simulink model "IEEE_9bus_4"  (Simulink 8.4)
settings: Solver=ode4  StartTime=0.0  StopTime=inf  FixedStep=Ts  RelTol=1e-3
PostLoadFcn:
  | Ts=25e-6;Rs=5*1.867;cs=1.4080e-004;
InitFcn:
  | Ts=25e-6;Rs=5*1.867;cs=1.4080e-004;
undefined symbols (not defined in the file): another_event_name, gcbh, my_event_name, sps_rtmsupport
libraries: spsVIMeasurementModel x36, powerlib x34, powerlib_meascontrol x18, rtlab x4, artemis x3, sps_avr x3
(part 1 of 3)
Description:
  | Model of a simple control system for use iin training.
settings Model: ARTEMISmethode_block_infos=$$__separator__$$IEEE_9bus_4/ARTEMIS Guide$$__separator__$$  Creator=Paul Baracos  LastModifiedBy=opal-user  BufferReuse=off
settings DataIOCC: SaveOutput=off  SaveTime=off  SignalLoggingName=sigsOut
settings OptimizationCC: BlockReduction=off  BooleanDataType=off  OptimizeBlockIOStorage=off  BufferReuse=off  GlobalBufferReuse=off  ExpressionFolding=off  ExpressionDepthLimit=128  LocalBlockOutputs=off  InitFltsAndDblsToZero=on
settings DebuggingCC: SaveWithParameterizedLinksMsg=none  SignalResolutionControl=TryResolveAllWithWarning  SolverPrmCheckMsg=none  MultiTaskDSMMsg=warning  MultiTaskCondExecSysMsg=none  StateNameClashWarn=none
settings HardwareCC: TargetUnknown=on
settings RTWCC: IncludeERTFirstTime=on
settings GRTTargetCC: TargetFcnLib=ansi_tfl_tmw.mat

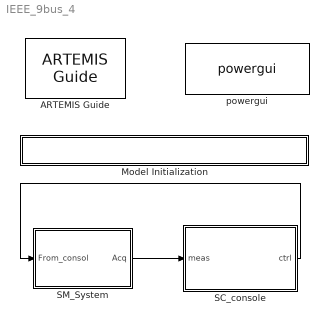
== system IEEE_9bus_4 ==
  ARTEMIS Guide : artemis/ARTEMIS/ARTEMIS Guide  Tag=FTSSmethode_opal_4hx0r99  Description=5.0_z1  lock=on  Ts=Ts  opt=art5  dyna=off  nb_perm=50  RT_fullcomp=off  ssn=off  ssn_itvc=off  ssn_ivic=off  ssn_ext=off  ssn_solver=Art5  ssn_impulse=off  ssn_quasimpulse=off  ssn_impulse_loop=2  paraExtinctionThy=off  Thy_Impulse=on  dtc=Off  dtc_opt=true impulse event detection  ao=on  simtype=off  ct_mac=off  lin_mov=off  lsp=[0.001 2]  spike_skip=Disabled  dtc_extra=1  dtc_sws=normal  dtc_pied=0.5  SPSRulesBlock=SPSRules  tre=on  ctmm=off  LF=off  dpl_type=ARTEMiS DPL  rlc_type=off  custom_type=off  para=off  ssn_ImpulseLoopBlockedStateUpdate=2  ssn_mov_iter_number=5  ssn_switch_iter_number=5
  Model Initialization : Subsystem  mask(Model Functions){InitFcnX=Ts=25e-6;Rs=5*1.867;cs=1.4080e-004;, prel=off, posl=on, inif=on, strf=off}
      mask prompts: InitFcnX "Initialisation"; prel "Preload Function"; posl "PostLoad Function"; inif "InitFcn"; strf "StartFcn"
      mask init:
      | currentBlock = gcb;
      | root = bdroot(currentBlock);
      | 
      | if ~strcmp(get_param(root,'BlockDiagramType'),'library')
      |     if prel==1
      |         set_param(root, 'PreLoadFcn', InitFcnX);
      |     else
      |         set_param(root, 'PreLoadFcn', '');
      |     end
      |     if inif==1
      |         set_param(root, 'InitFcn', InitFcnX);
      |     else
      |         set_param(root, 'InitFcn', '');
      |     end
      |     if strf==1
      |         set_param(root, 'StartFcn', InitFcnX);
      |     else
      |         set_param(root, 'StartFcn', '');
      |     end
      |     if posl==1
      |         set_param(root, 'PostLoadFcn', InitFcnX);
      |     else
      |         set_param(root, 'PostLoadFcn', '');
      |     end
      | end
      | 
      | pos = get_param(currentBlock, 'Position');
      | width = pos(3) - pos(1); height = pos(4) - pos(2);
      | txt = [ upper(root) '\n' '- InitFcn. . . . . '  get_param(root, 'InitFcn') ];
      settings: CopyFcn=set_param(gcb,'LinkStatus','none')
      mask Display: text(5, height*0.5, txt, 'horizontalAlignment', 'left', 'verticalAlignment', 'middle') ;
  SC_console : Subsystem
  SM_System : Subsystem
  powergui : powerlib/powergui  Priority=1  SimulationMode=Discrete  SolverType=Tustin  SampleTime=Ts  frequency=60  SPID=off  DisableSnubberDevices=off  DisableRonSwitches=off  DisableVfSwitches=off  SwTol=0  DisplayEquations=off  Interpol=off  methode=off  Ts=0  frequencyindice=60  Pbase=100e6  ErrMax=1e-4  Iterations=50  UnitsV=kV  UnitsW=MW  FunctionMessages=off  echomessages=off  HookPort=off  EnableUseOfTLC=off  x0status=steady  RestoreLinks=warning  ResistiveCurrentMeasurement=off  Frange=[0:2:500]  Ylog=off  Xlog=on  ShowGrid=off  save=off  variable=ZData  structure=0  ZoomFFT=on  StartTime=0.0  cycles=1  DisplayStyle=1  fundamental=60  FreqAxis=off  MaxFrequency=1000  frequencyindicesteady=1  RmsSteady=1  display=off
  wires:
  SC_console/1(ctrl) -> SM_System/1(From_consol)
  SM_System/1(Acq) -> SC_console/1(meas)

== system IEEE_9bus_4/Model Initialization ==

== system IEEE_9bus_4/SC_console ==
  note: System Setting
  note: Green for basic setting/scoping
  note: Orange for advanced setting/scoping
  note: System Scoping
  note: 7-Three-Phase Bus Transmission and Distribution System
  meas : Inport
  Breakers Control1 : Subsystem
  Fault Set1 : Subsystem  mask(fault set){Tacq=1, Tst=[0.5 0 10], Tdr=[0.1 0 10], Ftype=0:no fault, L1=off, L2=off, L3=off}
      mask prompts: Tacq "acquisition period"; Tst "fault start time set [Tst, Tst_var, Tst_pd]"; Tdr "fault duration set [Tst, Tst_var, Tst_pd]"; Ftype "fault_type"; L1 "Location 1"; L2 "Location 2"; L3 "Location 3"
      mask help:
      | output dimention: 8=1+3+3+1
      |
      | acquisition period, Tacq
      |
      | fault start time set [Tst, Tst_var, Tst_pd]
      | if Tst_var=0, fault starts at Tst
      | if Tst_var<>0, Tst varies from Tst to Tst+Tst_var, variation cycle is Tst_pd.
      |
      | fault duration set [Tdr, Tdr_var, Tdr_pd]
      | if Tdr_var=0, fault durstion is fixed, equal Tdr
      | if Tdr_var<>0, fault duration varies from Tdr to Tdr+Tdr_var, variation cycle is Tdr_pd.
      |
      | fault_type
      mask init:
      | switch Ftype
      |     case 1
      |         x='no fault';
      |     case 2
      | 	x='a fault';
      |     case 3
      | 	x='b fault';
      |     case 4
      | 	x='c fault';
      |     case 5
      | 	x='ab fault';
      |     case 6
      | 	x='ac fault';
      |     case 7
      | 	x='bc fault';
      |     case 8
      | 	x='abc gnd fault';
      | end
      mask TypeOptions Ftype: 0:no fault | 1:a fault | 2: b fault | 3:c fault | 4:ab fault | 5: ac fault | 6: bc fault | 7:abc-gnd fault
      mask Display: disp(x,Tacq)
  Help : artemis/Internal/Help  docfile=..\help\adgrid22_7bus_hvac.html
  Mux : Mux  Inputs=3
  OpComm1 : rtlab/OpComm  nbport=1  groupe_acq=1  subsys_rate=0  st=0  Synchronization=on  Interpolation=on  Threshold=1.0  Missed_Data=off  Sim_Time=off  Samples=off  dynSigOut=off  from_console=0  warning_done=off  writeOpCommFile=off  Offset=off
  SM_Select : Subsystem
  Subsystem : Subsystem
  www.opal-rt.com1 : artemis/Internal/www.opal-rt.com  SystemSampleTime=-1
  ctrl : Outport
  wires:
  meas/1 -> OpComm1/1
  Mux/1 -> ctrl/1
  Fault Set1/1(Out1) -> Mux/2
  Breakers Control1/1(BR_CTRL) -> Mux/1
  SM_Select/1(SM) -> Mux/3
  OpComm1/1 -> Subsystem/1(In3)

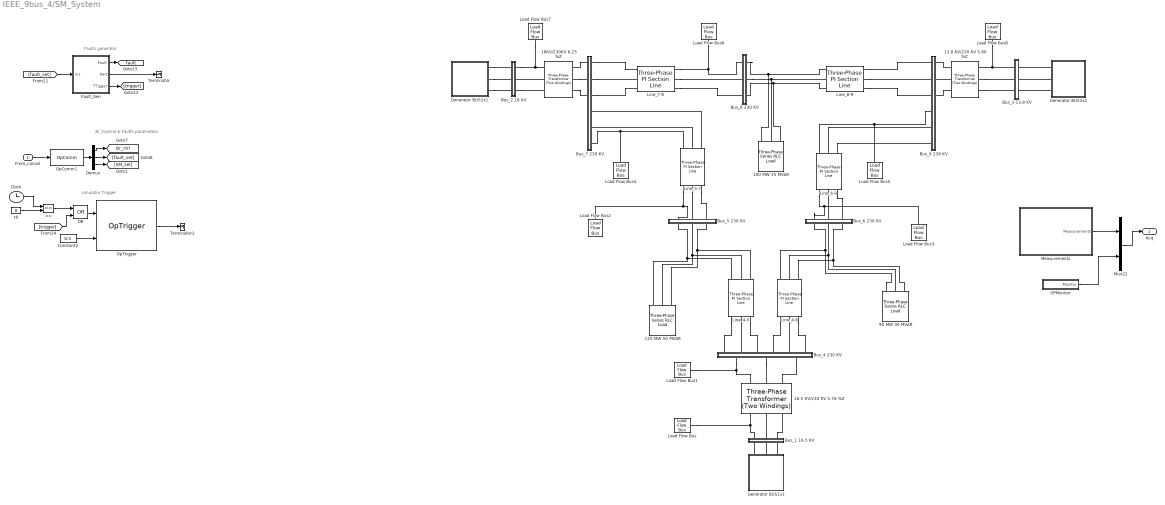
== system IEEE_9bus_4/SM_System ==
  note: Br_Control & Faults parameters
  note: Faults generator
  note: simulator Trigger
  From_consol : Inport
  100 MW 35 MVAR : powerlib/Elements/Three-Phase Series RLC Load  LConnTagsString=A|B|C  Configuration=Y (grounded)  NominalVoltage=(230000)*1.01601  NominalFrequency=60  ActivePower=100e6  InductivePower=35e6  CapacitivePower=0  Measurements=Branch voltages and currents  LoadType=constant PQ
  125 MW 50 MVAR : powerlib/Elements/Three-Phase Series RLC Load  LConnTagsString=A|B|C  Configuration=Y (grounded)  NominalVoltage=(230000)*0.996126  NominalFrequency=60  ActivePower=125e6  InductivePower=50e6  CapacitivePower=0  Measurements=Branch voltages and currents  LoadType=constant PQ
  13.8 KV/230 KV 5.86 %Z : powerlib/Elements/Three-Phase Transformer (Two Windings)  Winding1Connection=Yg  UNITS=pu  NominalPower=[ 128e6 , 60 ]  Winding1=[ 13.8e3 , 1e-6 , 0.0 ]  Winding2Connection=Yg  Winding2=[ 230e3 , 1e-6, 0.075008 ]  SetSaturation=off  Rm=inf  Lm=inf  Saturation=[ 0,0 ; 0.0024,1.2 ; 1.0,1.52 ]  Hysteresis=off  DataFile='hysteresis'  SetInitialFlux=off  InitialFluxes=[ 0.8 , -0.8 , 0.7 ]  Measurements=None  MoreParameters=off  BreakLoop=off  DataType=off  TransfoNumber=1
  "16.5 KV/230 KV 5.76 %Z     " : powerlib/Elements/Three-Phase Transformer (Two Windings)  Winding1Connection=Yg  UNITS=pu  NominalPower=[ 247.5e6 , 60 ]  Winding1=[ 16.5e3 , 1e-6, 0.0 ]  Winding2Connection=Yg  Winding2=[ 230e3 ,1e-6, 0.14256 ]  SetSaturation=off  Rm=inf  Lm=inf  Saturation=[ 0,0 ; 0.0024,1.2 ; 1.0,1.52 ]  Hysteresis=off  DataFile='hysteresis'  SetInitialFlux=off  InitialFluxes=[ 0.8 , -0.8 , 0.7 ]  Measurements=None  MoreParameters=off  BreakLoop=off  DataType=off  TransfoNumber=1
  18KV/230KV 6.25 %Z : powerlib/Elements/Three-Phase Transformer (Two Windings)  Winding1Connection=Yg  UNITS=pu  NominalPower=[ 192e6 , 60 ]  Winding1=[ 18e3 , 1e-6 , 0.0 ]  Winding2Connection=Yg  Winding2=[ 230e3 , 1e-6, 0.12 ]  SetSaturation=off  Rm=inf  Lm=inf  Saturation=[ 0,0 ; 0.0024,1.2 ; 1.0,1.52 ]  Hysteresis=off  DataFile='hysteresis'  SetInitialFlux=off  InitialFluxes=[ 0.8 , -0.8 , 0.7 ]  Measurements=None  MoreParameters=off  BreakLoop=off  DataType=off  TransfoNumber=1
  90 MW 30 MVAR : powerlib/Elements/Three-Phase Series RLC Load  LConnTagsString=A|B|C  Configuration=Y (grounded)  NominalVoltage=(230000)*1.01311  NominalFrequency=60  ActivePower=90e6  InductivePower=30e6  CapacitivePower=0  Measurements=Branch voltages and currents  LoadType=constant PQ
  == : RelationalOperator  Operator===  InputSameDT=on
  Bus_1 16.5 KV : Subsystem  DialogController=POWERSYS.PowerSysDialog  LoadFcn=sps_rtmsupport('LoadFcn',gcbh);  StartFcn=sps_rtmsupport('StartFcn',gcbh);  StopFcn=sps_rtmsupport('StopFcn',gcbh);  mask(Three-Phase VI Measurement){VoltageMeasurement=phase-to-phase, SetLabelV=on, LabelV=Vabc_1, Vpu=off, VpuLL=off, CurrentMeasurement=yes, SetLabelI=on, LabelI=Iabc_1, Ipu=off, Pbase=100e6, Vbase=16.5e3, OutputType=Complex, PhasorSimulation=off, PSBequivalent=0}
      mask prompts: VoltageMeasurement "Voltage measurement"; SetLabelV "Use a label"; LabelV "Signal label  (use a From block to collect this signal)"; Vpu "Voltages in pu,  based on peak value of nominal phase-to-ground voltage"; VpuLL "Voltages in pu,  based on peak value of nominal phase-to-phase  voltage"; CurrentMeasurement "Current measurement"; SetLabelI "Use a label"; LabelI "Signal label  (use a From block to collect this signal)"; Ipu "Currents in pu"; Pbase "Base power ( VA 3 phase)"; Vbase "Nominal voltage used for pu measurement (Vrms phase-phase) :"; OutputType "Output signals in:"; PhasorSimulation "Phasor simulation (internal use)"; PSBequivalent "Equivalent circuit (internal use)"
      mask help:
      | Ideal three-phase voltage and current measurements.
      |
      | The block can output the voltages and currents in per unit values or in volts and amperes.
      mask init:
      | block = gcb;
      | Kv=1;
      | Ki=1;
      | [Kv,Ki] = powericon('ThreePhaseVIMeasurementParam',block,Vpu,VpuLL,Ipu,Vbase,Pbase,PhasorSimulation,OutputType);
      | powericon('ThreePhaseVIMeasurementCback',block);
      | power_initmask();
      settings: CopyFcn=sps_rtmsupport('CopyFcn',gcbh); powericon('ThreePhaseVIMeasurementCopy',gcb)  DeleteFcn=sps_rtmsupport('DeleteFcn',gcbh);  UndoDeleteFcn=sps_rtmsupport('UndoDeleteFcn',gcbh);  ModelCloseFcn=sps_rtmsupport('ModelCloseFcn',gcbh);  PreSaveFcn="sps_rtmsupport('PreSaveFcn',gcbh);  set_param(gcb,'LinkStatus','restore')"  PostSaveFcn=sps_rtmsupport('PostSaveFcn',gcbh);  NameChangeFcn=sps_rtmsupport('NameChangeFcn',gcbh);  PreCopyFcn=sps_rtmsupport('PreCopyFcn',gcbh);  OpenFcn=sps_rtmsupport('OpenFcn',gcbh, [1 2 4 5 6 7 9 -12 13]);  CloseFcn=sps_rtmsupport('CloseFcn',gcbh);  PreDeleteFcn=sps_rtmsupport('PreDeleteFcn',gcbh);
      mask Help: helpview(psbhelp)
      mask TypeOptions VoltageMeasurement: no | phase-to-ground | phase-to-phase
      mask Callback VoltageMeasurement: powericon('ThreePhaseVIMeasurementCback',gcb,'Vselector');
      mask Callback SetLabelV: powericon('ThreePhaseVIMeasurementCback',gcb,'');
      mask Callback Vpu: powericon('ThreePhaseVIMeasurementCback',gcb,'Vpu');
      mask Callback VpuLL: powericon('ThreePhaseVIMeasurementCback',gcb,'VpuLL');
      mask TypeOptions CurrentMeasurement: no | yes
      mask Callback CurrentMeasurement: powericon('ThreePhaseVIMeasurementCback',gcb,'');
      mask Callback SetLabelI: powericon('ThreePhaseVIMeasurementCback',gcb,'');
      mask Callback LabelI: powericon('ThreePhaseVIMeasurementCback',gcb,'');
      mask Callback Ipu: powericon('ThreePhaseVIMeasurementCback',gcb,'');
      mask TypeOptions OutputType: Complex | Real-Imag | Magnitude-Angle | Magnitude
  Bus_2 18 KV : Subsystem  DialogController=POWERSYS.PowerSysDialog  LoadFcn=sps_rtmsupport('LoadFcn',gcbh);  StartFcn=sps_rtmsupport('StartFcn',gcbh);  StopFcn=sps_rtmsupport('StopFcn',gcbh);  mask(Three-Phase VI Measurement){VoltageMeasurement=phase-to-phase, SetLabelV=on, LabelV=Vabc_2, Vpu=off, VpuLL=off, CurrentMeasurement=yes, SetLabelI=on, LabelI=Iabc_2, Ipu=off, Pbase=100e6, Vbase=18e3, OutputType=Complex, PhasorSimulation=off, PSBequivalent=0}
      mask prompts: VoltageMeasurement "Voltage measurement"; SetLabelV "Use a label"; LabelV "Signal label  (use a From block to collect this signal)"; Vpu "Voltages in pu,  based on peak value of nominal phase-to-ground voltage"; VpuLL "Voltages in pu,  based on peak value of nominal phase-to-phase  voltage"; CurrentMeasurement "Current measurement"; SetLabelI "Use a label"; LabelI "Signal label  (use a From block to collect this signal)"; Ipu "Currents in pu"; Pbase "Base power ( VA 3 phase)"; Vbase "Nominal voltage used for pu measurement (Vrms phase-phase) :"; OutputType "Output signals in:"; PhasorSimulation "Phasor simulation (internal use)"; PSBequivalent "Equivalent circuit (internal use)"
      mask help:
      | Ideal three-phase voltage and current measurements.
      |
      | The block can output the voltages and currents in per unit values or in volts and amperes.
      mask init: same as IEEE_9bus_4/SM_System/Bus_1 16.5 KV
      settings: CopyFcn=sps_rtmsupport('CopyFcn',gcbh); powericon('ThreePhaseVIMeasurementCopy',gcb)  DeleteFcn=sps_rtmsupport('DeleteFcn',gcbh);  UndoDeleteFcn=sps_rtmsupport('UndoDeleteFcn',gcbh);  ModelCloseFcn=sps_rtmsupport('ModelCloseFcn',gcbh);  PreSaveFcn="sps_rtmsupport('PreSaveFcn',gcbh);  set_param(gcb,'LinkStatus','restore')"  PostSaveFcn=sps_rtmsupport('PostSaveFcn',gcbh);  NameChangeFcn=sps_rtmsupport('NameChangeFcn',gcbh);  PreCopyFcn=sps_rtmsupport('PreCopyFcn',gcbh);  OpenFcn=sps_rtmsupport('OpenFcn',gcbh, [1 2 4 5 6 7 9 -12 13]);  CloseFcn=sps_rtmsupport('CloseFcn',gcbh);  PreDeleteFcn=sps_rtmsupport('PreDeleteFcn',gcbh);
      mask Help: helpview(psbhelp)
      mask TypeOptions VoltageMeasurement: no | phase-to-ground | phase-to-phase
      mask Callback VoltageMeasurement: powericon('ThreePhaseVIMeasurementCback',gcb,'Vselector');
      mask Callback SetLabelV: powericon('ThreePhaseVIMeasurementCback',gcb,'');
      mask Callback Vpu: powericon('ThreePhaseVIMeasurementCback',gcb,'Vpu');
      mask Callback VpuLL: powericon('ThreePhaseVIMeasurementCback',gcb,'VpuLL');
      mask TypeOptions CurrentMeasurement: no | yes
      mask Callback CurrentMeasurement: powericon('ThreePhaseVIMeasurementCback',gcb,'');
      mask Callback SetLabelI: powericon('ThreePhaseVIMeasurementCback',gcb,'');
      mask Callback LabelI: powericon('ThreePhaseVIMeasurementCback',gcb,'');
      mask Callback Ipu: powericon('ThreePhaseVIMeasurementCback',gcb,'');
      mask TypeOptions OutputType: Complex | Real-Imag | Magnitude-Angle | Magnitude
  Bus_3 13.8 KV : Subsystem  DialogController=POWERSYS.PowerSysDialog  LoadFcn=sps_rtmsupport('LoadFcn',gcbh);  StartFcn=sps_rtmsupport('StartFcn',gcbh);  StopFcn=sps_rtmsupport('StopFcn',gcbh);  mask(Three-Phase VI Measurement){VoltageMeasurement=phase-to-phase, SetLabelV=on, LabelV=Vabc_3, Vpu=off, VpuLL=off, CurrentMeasurement=yes, SetLabelI=on, LabelI=Iabc_3, Ipu=off, Pbase=100e6, Vbase=13.8e3, OutputType=Complex, PhasorSimulation=off, PSBequivalent=0}
      mask prompts: VoltageMeasurement "Voltage measurement"; SetLabelV "Use a label"; LabelV "Signal label  (use a From block to collect this signal)"; Vpu "Voltages in pu,  based on peak value of nominal phase-to-ground voltage"; VpuLL "Voltages in pu,  based on peak value of nominal phase-to-phase  voltage"; CurrentMeasurement "Current measurement"; SetLabelI "Use a label"; LabelI "Signal label  (use a From block to collect this signal)"; Ipu "Currents in pu"; Pbase "Base power ( VA 3 phase)"; Vbase "Nominal voltage used for pu measurement (Vrms phase-phase) :"; OutputType "Output signals in:"; PhasorSimulation "Phasor simulation (internal use)"; PSBequivalent "Equivalent circuit (internal use)"
      mask help:
      | Ideal three-phase voltage and current measurements.
      |
      | The block can output the voltages and currents in per unit values or in volts and amperes.
      mask init: same as IEEE_9bus_4/SM_System/Bus_1 16.5 KV
      settings: CopyFcn=sps_rtmsupport('CopyFcn',gcbh); powericon('ThreePhaseVIMeasurementCopy',gcb)  DeleteFcn=sps_rtmsupport('DeleteFcn',gcbh);  UndoDeleteFcn=sps_rtmsupport('UndoDeleteFcn',gcbh);  ModelCloseFcn=sps_rtmsupport('ModelCloseFcn',gcbh);  PreSaveFcn="sps_rtmsupport('PreSaveFcn',gcbh);  set_param(gcb,'LinkStatus','restore')"  PostSaveFcn=sps_rtmsupport('PostSaveFcn',gcbh);  NameChangeFcn=sps_rtmsupport('NameChangeFcn',gcbh);  PreCopyFcn=sps_rtmsupport('PreCopyFcn',gcbh);  OpenFcn=sps_rtmsupport('OpenFcn',gcbh, [1 2 4 5 6 7 9 -12 13]);  CloseFcn=sps_rtmsupport('CloseFcn',gcbh);  PreDeleteFcn=sps_rtmsupport('PreDeleteFcn',gcbh);
      mask Help: helpview(psbhelp)
      mask TypeOptions VoltageMeasurement: no | phase-to-ground | phase-to-phase
      mask Callback VoltageMeasurement: powericon('ThreePhaseVIMeasurementCback',gcb,'Vselector');
      mask Callback SetLabelV: powericon('ThreePhaseVIMeasurementCback',gcb,'');
      mask Callback Vpu: powericon('ThreePhaseVIMeasurementCback',gcb,'Vpu');
      mask Callback VpuLL: powericon('ThreePhaseVIMeasurementCback',gcb,'VpuLL');
      mask TypeOptions CurrentMeasurement: no | yes
      mask Callback CurrentMeasurement: powericon('ThreePhaseVIMeasurementCback',gcb,'');
      mask Callback SetLabelI: powericon('ThreePhaseVIMeasurementCback',gcb,'');
      mask Callback LabelI: powericon('ThreePhaseVIMeasurementCback',gcb,'');
      mask Callback Ipu: powericon('ThreePhaseVIMeasurementCback',gcb,'');
      mask TypeOptions OutputType: Complex | Real-Imag | Magnitude-Angle | Magnitude
  Bus_4 230 KV : Subsystem
  Bus_5 230 KV : Subsystem  DialogController=POWERSYS.PowerSysDialog  LoadFcn=sps_rtmsupport('LoadFcn',gcbh);  StartFcn=sps_rtmsupport('StartFcn',gcbh);  StopFcn=sps_rtmsupport('StopFcn',gcbh);  mask(Three-Phase VI Measurement){VoltageMeasurement=phase-to-phase, SetLabelV=on, LabelV=Vabc_5, Vpu=off, VpuLL=off, CurrentMeasurement=yes, SetLabelI=on, LabelI=Iabc_5, Ipu=off, Pbase=100e6, Vbase=230e3, OutputType=Complex, PhasorSimulation=off, PSBequivalent=0}
      mask prompts: VoltageMeasurement "Voltage measurement"; SetLabelV "Use a label"; LabelV "Signal label  (use a From block to collect this signal)"; Vpu "Voltages in pu,  based on peak value of nominal phase-to-ground voltage"; VpuLL "Voltages in pu,  based on peak value of nominal phase-to-phase  voltage"; CurrentMeasurement "Current measurement"; SetLabelI "Use a label"; LabelI "Signal label  (use a From block to collect this signal)"; Ipu "Currents in pu"; Pbase "Base power ( VA 3 phase)"; Vbase "Nominal voltage used for pu measurement (Vrms phase-phase) :"; OutputType "Output signals in:"; PhasorSimulation "Phasor simulation (internal use)"; PSBequivalent "Equivalent circuit (internal use)"
      mask help:
      | Ideal three-phase voltage and current measurements.
      |
      | The block can output the voltages and currents in per unit values or in volts and amperes.
      mask init: same as IEEE_9bus_4/SM_System/Bus_1 16.5 KV
      settings: CopyFcn=sps_rtmsupport('CopyFcn',gcbh); powericon('ThreePhaseVIMeasurementCopy',gcb)  DeleteFcn=sps_rtmsupport('DeleteFcn',gcbh);  UndoDeleteFcn=sps_rtmsupport('UndoDeleteFcn',gcbh);  ModelCloseFcn=sps_rtmsupport('ModelCloseFcn',gcbh);  PreSaveFcn="sps_rtmsupport('PreSaveFcn',gcbh);  set_param(gcb,'LinkStatus','restore')"  PostSaveFcn=sps_rtmsupport('PostSaveFcn',gcbh);  NameChangeFcn=sps_rtmsupport('NameChangeFcn',gcbh);  PreCopyFcn=sps_rtmsupport('PreCopyFcn',gcbh);  OpenFcn=sps_rtmsupport('OpenFcn',gcbh, [1 2 4 5 6 7 9 -12 13]);  CloseFcn=sps_rtmsupport('CloseFcn',gcbh);  PreDeleteFcn=sps_rtmsupport('PreDeleteFcn',gcbh);
      mask Help: helpview(psbhelp)
      mask TypeOptions VoltageMeasurement: no | phase-to-ground | phase-to-phase
      mask Callback VoltageMeasurement: powericon('ThreePhaseVIMeasurementCback',gcb,'Vselector');
      mask Callback SetLabelV: powericon('ThreePhaseVIMeasurementCback',gcb,'');
      mask Callback Vpu: powericon('ThreePhaseVIMeasurementCback',gcb,'Vpu');
      mask Callback VpuLL: powericon('ThreePhaseVIMeasurementCback',gcb,'VpuLL');
      mask TypeOptions CurrentMeasurement: no | yes
      mask Callback CurrentMeasurement: powericon('ThreePhaseVIMeasurementCback',gcb,'');
      mask Callback SetLabelI: powericon('ThreePhaseVIMeasurementCback',gcb,'');
      mask Callback LabelI: powericon('ThreePhaseVIMeasurementCback',gcb,'');
      mask Callback Ipu: powericon('ThreePhaseVIMeasurementCback',gcb,'');
      mask TypeOptions OutputType: Complex | Real-Imag | Magnitude-Angle | Magnitude
  Bus_6 230 KV : Subsystem  DialogController=POWERSYS.PowerSysDialog  LoadFcn=sps_rtmsupport('LoadFcn',gcbh);  StartFcn=sps_rtmsupport('StartFcn',gcbh);  StopFcn=sps_rtmsupport('StopFcn',gcbh);  mask(Three-Phase VI Measurement){VoltageMeasurement=phase-to-phase, SetLabelV=on, LabelV=Vabc_6, Vpu=off, VpuLL=off, CurrentMeasurement=yes, SetLabelI=on, LabelI=Iabc_6, Ipu=off, Pbase=100e6, Vbase=230e3, OutputType=Complex, PhasorSimulation=off, PSBequivalent=0}
      mask prompts: VoltageMeasurement "Voltage measurement"; SetLabelV "Use a label"; LabelV "Signal label  (use a From block to collect this signal)"; Vpu "Voltages in pu,  based on peak value of nominal phase-to-ground voltage"; VpuLL "Voltages in pu,  based on peak value of nominal phase-to-phase  voltage"; CurrentMeasurement "Current measurement"; SetLabelI "Use a label"; LabelI "Signal label  (use a From block to collect this signal)"; Ipu "Currents in pu"; Pbase "Base power ( VA 3 phase)"; Vbase "Nominal voltage used for pu measurement (Vrms phase-phase) :"; OutputType "Output signals in:"; PhasorSimulation "Phasor simulation (internal use)"; PSBequivalent "Equivalent circuit (internal use)"
      mask help:
      | Ideal three-phase voltage and current measurements.
      |
      | The block can output the voltages and currents in per unit values or in volts and amperes.
      mask init: same as IEEE_9bus_4/SM_System/Bus_1 16.5 KV
      settings: CopyFcn=sps_rtmsupport('CopyFcn',gcbh); powericon('ThreePhaseVIMeasurementCopy',gcb)  DeleteFcn=sps_rtmsupport('DeleteFcn',gcbh);  UndoDeleteFcn=sps_rtmsupport('UndoDeleteFcn',gcbh);  ModelCloseFcn=sps_rtmsupport('ModelCloseFcn',gcbh);  PreSaveFcn="sps_rtmsupport('PreSaveFcn',gcbh);  set_param(gcb,'LinkStatus','restore')"  PostSaveFcn=sps_rtmsupport('PostSaveFcn',gcbh);  NameChangeFcn=sps_rtmsupport('NameChangeFcn',gcbh);  PreCopyFcn=sps_rtmsupport('PreCopyFcn',gcbh);  OpenFcn=sps_rtmsupport('OpenFcn',gcbh, [1 2 4 5 6 7 9 -12 13]);  CloseFcn=sps_rtmsupport('CloseFcn',gcbh);  PreDeleteFcn=sps_rtmsupport('PreDeleteFcn',gcbh);
      mask Help: helpview(psbhelp)
      mask TypeOptions VoltageMeasurement: no | phase-to-ground | phase-to-phase
      mask Callback VoltageMeasurement: powericon('ThreePhaseVIMeasurementCback',gcb,'Vselector');
      mask Callback SetLabelV: powericon('ThreePhaseVIMeasurementCback',gcb,'');
      mask Callback Vpu: powericon('ThreePhaseVIMeasurementCback',gcb,'Vpu');
      mask Callback VpuLL: powericon('ThreePhaseVIMeasurementCback',gcb,'VpuLL');
      mask TypeOptions CurrentMeasurement: no | yes
      mask Callback CurrentMeasurement: powericon('ThreePhaseVIMeasurementCback',gcb,'');
      mask Callback SetLabelI: powericon('ThreePhaseVIMeasurementCback',gcb,'');
      mask Callback LabelI: powericon('ThreePhaseVIMeasurementCback',gcb,'');
      mask Callback Ipu: powericon('ThreePhaseVIMeasurementCback',gcb,'');
      mask TypeOptions OutputType: Complex | Real-Imag | Magnitude-Angle | Magnitude
  Bus_7 230 KV : Subsystem
  Bus_8 230 KV : Subsystem  DialogController=POWERSYS.PowerSysDialog  LoadFcn=sps_rtmsupport('LoadFcn',gcbh);  StartFcn=sps_rtmsupport('StartFcn',gcbh);  StopFcn=sps_rtmsupport('StopFcn',gcbh);  mask(Three-Phase VI Measurement){VoltageMeasurement=phase-to-phase, SetLabelV=on, LabelV=Vabc_8, Vpu=off, VpuLL=off, CurrentMeasurement=yes, SetLabelI=on, LabelI=Iabc_8, Ipu=off, Pbase=100e6, Vbase=230e3, OutputType=Complex, PhasorSimulation=off, PSBequivalent=0}
      mask prompts: VoltageMeasurement "Voltage measurement"; SetLabelV "Use a label"; LabelV "Signal label  (use a From block to collect this signal)"; Vpu "Voltages in pu,  based on peak value of nominal phase-to-ground voltage"; VpuLL "Voltages in pu,  based on peak value of nominal phase-to-phase  voltage"; CurrentMeasurement "Current measurement"; SetLabelI "Use a label"; LabelI "Signal label  (use a From block to collect this signal)"; Ipu "Currents in pu"; Pbase "Base power ( VA 3 phase)"; Vbase "Nominal voltage used for pu measurement (Vrms phase-phase) :"; OutputType "Output signals in:"; PhasorSimulation "Phasor simulation (internal use)"; PSBequivalent "Equivalent circuit (internal use)"
      mask help:
      | Ideal three-phase voltage and current measurements.
      |
      | The block can output the voltages and currents in per unit values or in volts and amperes.
      mask init: same as IEEE_9bus_4/SM_System/Bus_1 16.5 KV
      settings: CopyFcn=sps_rtmsupport('CopyFcn',gcbh); powericon('ThreePhaseVIMeasurementCopy',gcb)  DeleteFcn=sps_rtmsupport('DeleteFcn',gcbh);  UndoDeleteFcn=sps_rtmsupport('UndoDeleteFcn',gcbh);  ModelCloseFcn=sps_rtmsupport('ModelCloseFcn',gcbh);  PreSaveFcn="sps_rtmsupport('PreSaveFcn',gcbh);  set_param(gcb,'LinkStatus','restore')"  PostSaveFcn=sps_rtmsupport('PostSaveFcn',gcbh);  NameChangeFcn=sps_rtmsupport('NameChangeFcn',gcbh);  PreCopyFcn=sps_rtmsupport('PreCopyFcn',gcbh);  OpenFcn=sps_rtmsupport('OpenFcn',gcbh, [1 2 4 5 6 7 9 -12 13]);  CloseFcn=sps_rtmsupport('CloseFcn',gcbh);  PreDeleteFcn=sps_rtmsupport('PreDeleteFcn',gcbh);
      mask Help: helpview(psbhelp)
      mask TypeOptions VoltageMeasurement: no | phase-to-ground | phase-to-phase
      mask Callback VoltageMeasurement: powericon('ThreePhaseVIMeasurementCback',gcb,'Vselector');
      mask Callback SetLabelV: powericon('ThreePhaseVIMeasurementCback',gcb,'');
      mask Callback Vpu: powericon('ThreePhaseVIMeasurementCback',gcb,'Vpu');
      mask Callback VpuLL: powericon('ThreePhaseVIMeasurementCback',gcb,'VpuLL');
      mask TypeOptions CurrentMeasurement: no | yes
      mask Callback CurrentMeasurement: powericon('ThreePhaseVIMeasurementCback',gcb,'');
      mask Callback SetLabelI: powericon('ThreePhaseVIMeasurementCback',gcb,'');
      mask Callback LabelI: powericon('ThreePhaseVIMeasurementCback',gcb,'');
      mask Callback Ipu: powericon('ThreePhaseVIMeasurementCback',gcb,'');
      mask TypeOptions OutputType: Complex | Real-Imag | Magnitude-Angle | Magnitude
  Bus_9 230 KV : Subsystem
  Clock : Clock
  Constant2 : Constant  Value=0.5
  Demux : Demux  Outputs=[14 11 1]
  Fault_Gen : Subsystem
  Generator BUS1x1 : Subsystem
  Generator BUS2x1 : Subsystem
  Generator BUS3x1 : Subsystem
  Line_4-5 : powerlib/Elements/Three-Phase PI Section Line  LConnTagsString=a|b|c  RConnTagsString=A|B|C  Frequency=60  Resistances=[ 0.0529 0.13225]  Inductances="[ 1.192e-3  2.38e-3]"  Capacitances=[8.82e-9 5.188e-9]  Length=100
  Line_4-6 : powerlib/Elements/Three-Phase PI Section Line  LConnTagsString=a|b|c  RConnTagsString=A|B|C  Frequency=60  Resistances=[ 0.08993 0.224825]  Inductances="[ 1.29e-3  3.22e-3]"  Capacitances=[7.922e-9 4.74e-9]  Length=100
  Line_5-7 : powerlib/Elements/Three-Phase PI Section Line  LConnTagsString=a|b|c  RConnTagsString=A|B|C  Frequency=60  Resistances=[ 0.16928 0.4232]  Inductances="[ 2.259e-3  5.64e-3]"  Capacitances=[15.34e-9 9.025e-9]  Length=100
  Line_6-9 : powerlib/Elements/Three-Phase PI Section Line  LConnTagsString=a|b|c  RConnTagsString=A|B|C  Frequency=60  Resistances=[ 0.20631 0.5157]  Inductances="[ 2.38e-3  6.09e-3]"  Capacitances=[17.95e-9 10.55e-9]  Length=100
  Line_7-8 : powerlib/Elements/Three-Phase PI Section Line  LConnTagsString=a|b|c  RConnTagsString=A|B|C  Frequency=60  Resistances=[0.044965 0.11241]  Inductances="[ 1.01e-3  2.02e-3]"  Capacitances=[7.471e-9 4.394e-9]  Length=100
  Line_8-9 : powerlib/Elements/Three-Phase PI Section Line  LConnTagsString=a|b|c  RConnTagsString=A|B|C  Frequency=60  Resistances=[ 0.062951 0.15737]  Inductances="[ 1.414e-3  3.53e-3]"  Capacitances=[10.47e-9 6.15e-9]  Length=100
  Load Flow Bus : powerlib/Measurements/Load Flow Bus  LConnTagsString=a  ID=BUS_1  Vbase=16.5e3  Vref=1.04  Vangle=0  VLF=1.04  angleLF=0
      settings: AttributesFormatString=%<ID>\n%<Vbase>V\n%<VLF>pu\n%<angleLF>deg.
  Load Flow Bus1 : powerlib/Measurements/Load Flow Bus  LConnTagsString=a  ID=BUS_4  Vbase=230e3  Vref=1  Vangle=0  VLF=1.026  angleLF=-2.214
      settings: AttributesFormatString=%<ID>\n%<Vbase>V\n%<VLF>pu\n%<angleLF>deg.
  Load Flow Bus2 : powerlib/Measurements/Load Flow Bus  LConnTagsString=a  ID=BUS_5  Vbase=230e3  Vref=1  Vangle=0  VLF=0.9961  angleLF=-3.98
      settings: AttributesFormatString=%<ID>\n%<Vbase>V\n%<VLF>pu\n%<angleLF>deg.
  Load Flow Bus3 : powerlib/Measurements/Load Flow Bus  LConnTagsString=a  ID=BUS_6  Vbase=230e3  Vref=1  Vangle=0  VLF=1.013  angleLF=-3.678
      settings: AttributesFormatString=%<ID>\n%<Vbase>V\n%<VLF>pu\n%<angleLF>deg.
  Load Flow Bus4 : powerlib/Measurements/Load Flow Bus  LConnTagsString=a  ID=BUS_7  Vbase=230e3  Vref=1  Vangle=0  VLF=1.026  angleLF=3.662
      settings: AttributesFormatString=%<ID>\n%<Vbase>V\n%<VLF>pu\n%<angleLF>deg.
  Load Flow Bus5 : powerlib/Measurements/Load Flow Bus  LConnTagsString=a  ID=BUS_9  Vbase=230e3  Vref=1  Vangle=0  VLF=1.032  angleLF=1.909
      settings: AttributesFormatString=%<ID>\n%<Vbase>V\n%<VLF>pu\n%<angleLF>deg.
  Load Flow Bus6 : powerlib/Measurements/Load Flow Bus  LConnTagsString=a  ID=BUS_8  Vbase=230e3  Vref=1  Vangle=0  VLF=1.016  angleLF=0.6755
      settings: AttributesFormatString=%<ID>\n%<Vbase>V\n%<VLF>pu\n%<angleLF>deg.
  Load Flow Bus7 : powerlib/Measurements/Load Flow Bus  LConnTagsString=a  ID=BUS_2  Vbase=18e3  Vref=1.025  Vangle=0  VLF=1.025  angleLF=9.222
      settings: AttributesFormatString=%<ID>\n%<Vbase>V\n%<VLF>pu\n%<angleLF>deg.
  Load Flow Bus8 : powerlib/Measurements/Load Flow Bus  LConnTagsString=a  ID=BUS_3  Vbase=13.8e3  Vref=1.025  Vangle=4.7  VLF=1.025  angleLF=4.606
      settings: AttributesFormatString=%<ID>\n%<Vbase>V\n%<VLF>pu\n%<angleLF>deg.
  Measurements : Subsystem
  Mux22 : Mux  Inputs=2
  OPMonitor : Subsystem
  OR : Logic  Operator=OR
  OpComm1 : rtlab/OpComm  nbport=1  groupe_acq=1  subsys_rate=Ts  st=Ts  Synchronization=on  Interpolation=on  Threshold=1.0  Missed_Data=off  Sim_Time=off  Samples=off  dynSigOut=off  from_console=1  warning_done=off  writeOpCommFile=off  Offset=off
  OpTrigger : rtlab/DataLogging/OpTrigger  Trig_Type=TRIGGER SIGNAL >= TRIGGER LEVEL  Trig_Offset=0  Acq_Group=1
  Terminator : Terminator
  Terminator2 : Terminator
  t0 : Constant  Value=0
  Acq : Outport
  tag scope: Br_ctrl=global, fault=global
  wires:
  From_consol/1 -> OpComm1/1
  OpComm1/1 -> Demux/1
  Demux/1 -> [Br_ctrl]
  Demux/2 -> [fault_set]
  Fault_Gen/3(TTigger) -> [trigger]
  Fault_Gen/2(Pert) -> Terminator/1
  [fault_set] -> Fault_Gen/1(In1)
  Fault_Gen/1(Fault) -> [fault]
  Constant2/1 -> OpTrigger/2
  OpTrigger/1 -> Terminator2/1
  Clock/1 -> ==/1
  t0/1 -> ==/2
  ==/1 -> OR/1
  [trigger] -> OR/2
  OR/1 -> OpTrigger/1
  Demux/3 -> [SM_sel]
  Mux22/1 -> Acq/1
  Measurements/1(Measurements) -> Mux22/1
  OPMonitor/1(Monitor) -> Mux22/2
  connections:
  18KV/230KV 6.25 %Z/LConn1 -- Bus_2 18 KV/RConn1 -- Load Flow Bus7/LConn1
  13.8 KV/230 KV 5.86 %Z/LConn1 -- Load Flow Bus8/LConn1 -- Bus_3 13.8 KV/LConn1
  "16.5 KV/230 KV 5.76 %Z     "/LConn1 -- Bus_1 16.5 KV/LConn1 -- Load Flow Bus/LConn1
  Load Flow Bus1/LConn1 -- Bus_4 230 KV/LConn1 -- "16.5 KV/230 KV 5.76 %Z     "/RConn1
  Bus_8 230 KV/LConn1 -- 100 MW 35 MVAR/LConn1 -- Line_8-9/LConn1
  Bus_8 230 KV/LConn2 -- 100 MW 35 MVAR/LConn2 -- Line_8-9/LConn2
  Line_8-9/LConn3 -- 100 MW 35 MVAR/LConn3 -- Bus_8 230 KV/LConn3
  Bus_5 230 KV/RConn1 -- 125 MW 50 MVAR/LConn1 -- Line_4-5/RConn1
  Bus_5 230 KV/RConn2 -- 125 MW 50 MVAR/LConn2 -- Line_4-5/RConn2
  Bus_5 230 KV/RConn3 -- 125 MW 50 MVAR/LConn3 -- Line_4-5/RConn3
  Bus_6 230 KV/RConn1 -- 90 MW 30 MVAR/LConn1 -- Line_4-6/RConn1
  Bus_6 230 KV/RConn2 -- 90 MW 30 MVAR/LConn2 -- Line_4-6/RConn2
  Bus_6 230 KV/RConn3 -- 90 MW 30 MVAR/LConn3 -- Line_4-6/RConn3
  Line_7-8/RConn1 -- Bus_8 230 KV/RConn1 -- Load Flow Bus6/LConn1
  Line_5-7/LConn1 -- Load Flow Bus2/LConn1 -- Bus_5 230 KV/LConn1
  Bus_7 230 KV/RConn6 -- Load Flow Bus4/LConn1 -- Line_5-7/RConn1
  Bus_9 230 KV/LConn4 -- Load Flow Bus5/LConn1 -- Line_6-9/RConn1
  Load Flow Bus3/LConn1 -- Bus_6 230 KV/LConn1 -- Line_6-9/LConn1
  Generator BUS2x1/RConn1 -- Bus_2 18 KV/LConn1
  Generator BUS2x1/RConn3 -- Bus_2 18 KV/LConn3
  Generator BUS3x1/RConn3 -- Bus_3 13.8 KV/RConn3
  Generator BUS3x1/RConn2 -- Bus_3 13.8 KV/RConn2
  Generator BUS3x1/RConn1 -- Bus_3 13.8 KV/RConn1
  Line_4-6/LConn3 -- Bus_4 230 KV/RConn6
  Line_4-6/LConn1 -- Bus_4 230 KV/RConn4
  Line_4-6/LConn2 -- Bus_4 230 KV/RConn5
  Line_4-5/LConn3 -- Bus_4 230 KV/RConn3
  Line_4-5/LConn1 -- Bus_4 230 KV/RConn1
  Line_4-5/LConn2 -- Bus_4 230 KV/RConn2
  Line_6-9/RConn3 -- Bus_9 230 KV/LConn6
  Line_6-9/LConn3 -- Bus_6 230 KV/LConn3
  Line_6-9/LConn2 -- Bus_6 230 KV/LConn2
  Line_6-9/RConn2 -- Bus_9 230 KV/LConn5
  Line_5-7/RConn3 -- Bus_7 230 KV/RConn4
  Line_5-7/RConn2 -- Bus_7 230 KV/RConn5
  Line_5-7/LConn3 -- Bus_5 230 KV/LConn3
  Line_5-7/LConn2 -- Bus_5 230 KV/LConn2
  Line_8-9/RConn3 -- Bus_9 230 KV/LConn3
  Line_8-9/RConn1 -- Bus_9 230 KV/LConn1
  Line_8-9/RConn2 -- Bus_9 230 KV/LConn2
  Line_7-8/RConn3 -- Bus_8 230 KV/RConn3
  Line_7-8/RConn2 -- Bus_8 230 KV/RConn2
  Bus_7 230 KV/RConn3 -- Line_7-8/LConn3
  Bus_7 230 KV/RConn2 -- Line_7-8/LConn2
  Bus_7 230 KV/RConn1 -- Line_7-8/LConn1
  "16.5 KV/230 KV 5.76 %Z     "/RConn3 -- Bus_4 230 KV/LConn3
  Bus_4 230 KV/LConn2 -- "16.5 KV/230 KV 5.76 %Z     "/RConn2
  13.8 KV/230 KV 5.86 %Z/RConn3 -- Bus_9 230 KV/RConn3
  13.8 KV/230 KV 5.86 %Z/RConn2 -- Bus_9 230 KV/RConn2
  13.8 KV/230 KV 5.86 %Z/RConn1 -- Bus_9 230 KV/RConn1
  Bus_1 16.5 KV/LConn2 -- "16.5 KV/230 KV 5.76 %Z     "/LConn2
  Bus_1 16.5 KV/LConn3 -- "16.5 KV/230 KV 5.76 %Z     "/LConn3
  Generator BUS1x1/RConn3 -- Bus_1 16.5 KV/RConn3
  Generator BUS1x1/RConn2 -- Bus_1 16.5 KV/RConn2
  Generator BUS1x1/RConn1 -- Bus_1 16.5 KV/RConn1
  13.8 KV/230 KV 5.86 %Z/LConn3 -- Bus_3 13.8 KV/LConn3
  13.8 KV/230 KV 5.86 %Z/LConn2 -- Bus_3 13.8 KV/LConn2
  18KV/230KV 6.25 %Z/RConn3 -- Bus_7 230 KV/LConn3
  Bus_7 230 KV/LConn1 -- 18KV/230KV 6.25 %Z/RConn1
  Bus_2 18 KV/RConn3 -- 18KV/230KV 6.25 %Z/LConn3
  18KV/230KV 6.25 %Z/RConn2 -- Bus_7 230 KV/LConn2
  18KV/230KV 6.25 %Z/LConn2 -- Bus_2 18 KV/RConn2
  Generator BUS2x1/RConn2 -- Bus_2 18 KV/LConn2

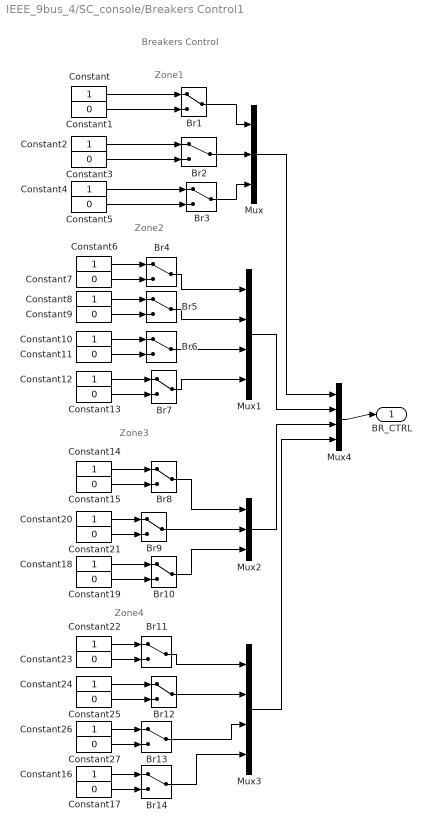
== system IEEE_9bus_4/SC_console/Breakers Control1 ==
  note: Zone1
  note: Zone4
  note: Zone2
  note: Zone3
  note: Breakers Control
  Br{1..14} (14 alike) : ManualSwitch
  Constant{,2,4,6,8,10,12,14,16,18,20,22,24,26} (14 alike) : Constant
  Constant{1,3,5,7,9,11,13,15,17,19,21,23,25,27} (14 alike) : Constant  Value=0
  Mux : Mux  Inputs=3
  Mux1 : Mux
  Mux2 : Mux  Inputs=3
  Mux3 : Mux
  Mux4 : Mux
  BR_CTRL : Outport
  wires:
  Constant/1 -> Br1/1
  Constant1/1 -> Br1/2
  Constant2/1 -> Br2/1
  Constant3/1 -> Br2/2
  Constant4/1 -> Br3/1
  Constant5/1 -> Br3/2
  Constant6/1 -> Br4/1
  Constant7/1 -> Br4/2
  Constant8/1 -> Br5/1
  Constant9/1 -> Br5/2
  Constant10/1 -> Br6/1
  Constant11/1 -> Br6/2
  Constant12/1 -> Br7/1
  Constant13/1 -> Br7/2
  Constant14/1 -> Br8/1
  Constant15/1 -> Br8/2
  Constant18/1 -> Br10/1
  Constant19/1 -> Br10/2
  Constant20/1 -> Br9/1
  Constant21/1 -> Br9/2
  Constant22/1 -> Br11/1
  Constant23/1 -> Br11/2
  Constant24/1 -> Br12/1
  Constant25/1 -> Br12/2
  Constant26/1 -> Br13/1
  Constant27/1 -> Br13/2
  Br1/1 -> Mux/1
  Br2/1 -> Mux/2
  Br3/1 -> Mux/3
  Br4/1 -> Mux1/1
  Br5/1 -> Mux1/2
  Br6/1 -> Mux1/3
  Br7/1 -> Mux1/4
  Br8/1 -> Mux2/1
  Br9/1 -> Mux2/2
  Br10/1 -> Mux2/3
  Br11/1 -> Mux3/1
  Br12/1 -> Mux3/2
  Br13/1 -> Mux3/3
  Mux2/1 -> Mux4/3
  Mux3/1 -> Mux4/4
  Mux/1 -> Mux4/1
  Mux1/1 -> Mux4/2
  Br14/1 -> Mux3/4
  Constant16/1 -> Br14/1
  Constant17/1 -> Br14/2
  Mux4/1 -> BR_CTRL/1

== system IEEE_9bus_4/SC_console/Fault Set1 ==
  Constant : Constant  Value=Ftype-1
  Constant1 : Constant  Value=L1
  Constant2 : Constant  Value=L2
  Constant3 : Constant  Value=L3
  Mux1 : Mux  Inputs=[1 3 3 1 1 1 1]
  Tacq : Constant  Value=Tacq
  Tdrp : Constant  Value=Tdr
  Tstp : Constant  Value=Tst
  Out1 : Outport  InitialOutput=0
  wires:
  Tacq/1 -> Mux1/1
  Tstp/1 -> Mux1/2
  Tdrp/1 -> Mux1/3
  Mux1/1 -> Out1/1
  Constant/1 -> Mux1/4
  Constant1/1 -> Mux1/5
  Constant2/1 -> Mux1/6
  Constant3/1 -> Mux1/7

== system IEEE_9bus_4/SC_console/SM_Select ==
  note: SM1: 1
      | SM2: 2
      | SM3: 3
      | SM4: 4
      | SM5: 5
  note: Select Machine for scop
  Machine_Select : Constant  Value=2
  SM : Outport
  wires:
  Machine_Select/1 -> SM/1

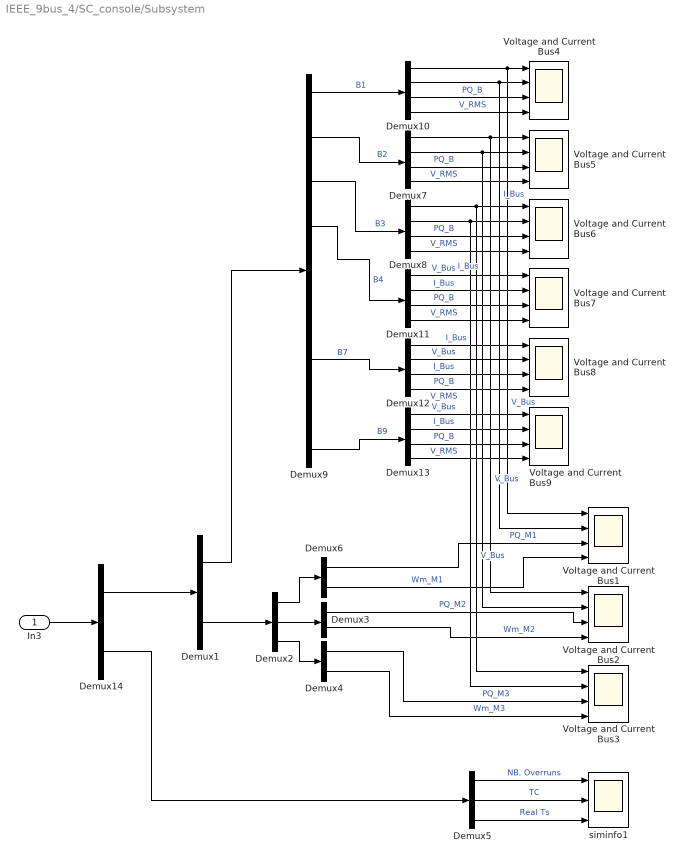
== system IEEE_9bus_4/SC_console/Subsystem ==
  In3 : Inport
  Demux1 : Demux  Outputs=[99 9]
  Demux{7..8,10..13} (6 alike) : Demux  Outputs=[3 3 2 3]
  Demux14 : Demux  Outputs=[108 3]
  Demux2 : Demux  Outputs=3
  Demux3 : Demux  Outputs=[2 1]
  Demux4 : Demux  Outputs=[2 1]
  Demux5 : Demux  Outputs=3
  Demux6 : Demux  Outputs=[2 1]
  Demux9 : Demux  Outputs=[11 11 11 11 11 11 11 11 11]
  Voltage and Current Bus{1..9} (9 alike) : Scope  NumInputPorts=4
      Voltage and Current Bus1 settings: TimeRange=0.1  YMin=-1.25~-0.75~-0.5~1  YMax=1.25~0.75~0.3~1.00001  SaveName=mach10  MaxDataPoints=15000
      Voltage and Current Bus2 settings: TimeRange=0.1  YMin=-1.25~-0.75~-0.5~1  YMax=1.25~0.75~0.3~1.00001  SaveName=mach11  MaxDataPoints=15000
      Voltage and Current Bus3 settings: TimeRange=0.1  YMin=-1.25~-0.75~-0.5~1  YMax=1.25~0.75~0.3~1.00001  SaveName=mach12  MaxDataPoints=15000
      Voltage and Current Bus4 settings: TimeRange=0.1  YMin=-1~-0.9~-0.8~-5  YMax=1~0.9~0.5~5  SaveName=mach13  MaxDataPoints=15000
      Voltage and Current Bus5 settings: TimeRange=0.1  YMin=-1~-0.9~-0.8~-5  YMax=1~0.9~0.5~5  SaveName=mach  MaxDataPoints=15000
      Voltage and Current Bus6 settings: TimeRange=0.1  YMin=-1~-0.9~-0.8~-5  YMax=1~0.9~0.5~5  SaveName=mach1  MaxDataPoints=15000
      Voltage and Current Bus7 settings: TimeRange=0.1  YMin=-1~-0.9~-0.8~-5  YMax=1~0.9~0.5~5  SaveName=mach3  MaxDataPoints=15000
      Voltage and Current Bus8 settings: TimeRange=0.1  YMin=-1~-0.9~-0.8~-5  YMax=1~0.9~0.5~5  SaveName=mach4  MaxDataPoints=15000
      Voltage and Current Bus9 settings: TimeRange=0.1  YMin=-1~-0.9~-0.8~-5  YMax=1~0.9~0.5~5  SaveName=mach5  MaxDataPoints=15000
  siminfo1 : Scope  NumInputPorts=3
      settings: TimeRange=0.8  YMin=-1~-1~-1  YMax=1~1~1  SaveName=mach2  MaxDataPoints=15000
  wires:
  Demux5/3 -> siminfo1/3  "Real Ts"
  Demux5/1 -> siminfo1/1  "NB. Overruns"
  Demux5/2 -> siminfo1/2  "TC"
  Demux3/2 -> Voltage and Current Bus2/4  "Wm_M2"
  Demux2/1 -> Demux6/1
  Demux6/1 -> Voltage and Current Bus1/3  "PQ_M1"
  Demux1/2 -> Demux2/1
  Demux4/2 -> Voltage and Current Bus3/4  "Wm_M3"
  Demux4/1 -> Voltage and Current Bus3/3  "PQ_M3"
  Demux3/1 -> Voltage and Current Bus2/3  "PQ_M2"
  Demux2/2 -> Demux3/1
  Demux2/3 -> Demux4/1
  Demux6/2 -> Voltage and Current Bus1/4  "Wm_M1"
  Demux1/1 -> Demux9/1
  Demux9/1 -> Demux10/1  "B1"
  Demux10/1 -> Voltage and Current Bus1/1, Voltage and Current Bus4/1  "V_Bus"
  Demux10/2 -> Voltage and Current Bus1/2, Voltage and Current Bus4/2  "I_Bus"
  Demux10/3 -> Voltage and Current Bus4/3  "PQ_B"
  In3/1 -> Demux14/1
  Demux14/2 -> Demux5/1
  Demux14/1 -> Demux1/1
  Demux10/4 -> Voltage and Current Bus4/4  "V_RMS"
  Demux7/1 -> Voltage and Current Bus2/1, Voltage and Current Bus5/1  "V_Bus"
  Demux7/2 -> Voltage and Current Bus2/2, Voltage and Current Bus5/2  "I_Bus"
  Demux7/3 -> Voltage and Current Bus5/3  "PQ_B"
  Demux7/4 -> Voltage and Current Bus5/4  "V_RMS"
  Demux8/1 -> Voltage and Current Bus3/1, Voltage and Current Bus6/1  "V_Bus"
  Demux8/2 -> Voltage and Current Bus3/2, Voltage and Current Bus6/2  "I_Bus"
  Demux8/3 -> Voltage and Current Bus6/3  "PQ_B"
  Demux8/4 -> Voltage and Current Bus6/4  "V_RMS"
  Demux11/1 -> Voltage and Current Bus7/1  "V_Bus"
  Demux11/2 -> Voltage and Current Bus7/2  "I_Bus"
  Demux11/3 -> Voltage and Current Bus7/3  "PQ_B"
  Demux11/4 -> Voltage and Current Bus7/4  "V_RMS"
  Demux12/1 -> Voltage and Current Bus8/1  "V_Bus"
  Demux12/2 -> Voltage and Current Bus8/2  "I_Bus"
  Demux12/3 -> Voltage and Current Bus8/3  "PQ_B"
  Demux12/4 -> Voltage and Current Bus8/4  "V_RMS"
  Demux13/1 -> Voltage and Current Bus9/1  "V_Bus"
  Demux13/2 -> Voltage and Current Bus9/2  "I_Bus"
  Demux13/3 -> Voltage and Current Bus9/3  "PQ_B"
  Demux13/4 -> Voltage and Current Bus9/4  "V_RMS"
  Demux9/2 -> Demux7/1  "B2"
  Demux9/3 -> Demux8/1  "B3"
  Demux9/4 -> Demux11/1  "B4"
  Demux9/7 -> Demux12/1  "B7"
  Demux9/9 -> Demux13/1  "B9"

== system IEEE_9bus_4/SM_System/Bus_1 16.5 KV ==
  Kv : Gain  Gain=Ki  SaturateOnIntegerOverflow=on  OutDataTypeStr=Inherit: Same as input  ParamDataTypeStr=Inherit: Same as input
  Kv1 : Gain  Gain=Kv  SaturateOnIntegerOverflow=on  OutDataTypeStr=Inherit: Same as input  ParamDataTypeStr=Inherit: Same as input
  Mode I : spsVIMeasurementModel/Complex
  Mode V : spsVIMeasurementModel/Complex
  Model : spsVIMeasurementModel/VI_phase  SystemSampleTime=-1
  A : PMIOPort  Port=1  Side=Left
  B : PMIOPort  Port=2  Side=Left
  C : PMIOPort  Port=3  Side=Left
  a : PMIOPort  Port=4  Side=Right
  b : PMIOPort  Port=5  Side=Right
  c : PMIOPort  Port=6  Side=Right
  tag scope: Iabc_1=global, Vabc_1=global
  wires:
  Model/2 -> Kv/1
  Model/1 -> Kv1/1
  Kv/1 -> Mode I/1
  Kv1/1 -> Mode V/1
  Mode I/1 -> [Iabc_1]
  Mode V/1 -> [Vabc_1]
  connections:
  Model/RConn3 -- c/RConn1
  Model/RConn1 -- a/RConn1
  Model/RConn2 -- b/RConn1
  Model/LConn3 -- C/RConn1
  Model/LConn1 -- A/RConn1
  Model/LConn2 -- B/RConn1

== system IEEE_9bus_4/SM_System/Bus_2 18 KV ==
  Kv : Gain  Gain=Ki  SaturateOnIntegerOverflow=on  OutDataTypeStr=Inherit: Same as input  ParamDataTypeStr=Inherit: Same as input
  Kv1 : Gain  Gain=Kv  SaturateOnIntegerOverflow=on  OutDataTypeStr=Inherit: Same as input  ParamDataTypeStr=Inherit: Same as input
  Mode I : spsVIMeasurementModel/Complex
  Mode V : spsVIMeasurementModel/Complex
  Model : spsVIMeasurementModel/VI_phase  SystemSampleTime=-1
  A : PMIOPort  Port=1  Side=Left
  B : PMIOPort  Port=2  Side=Left
  C : PMIOPort  Port=3  Side=Left
  a : PMIOPort  Port=4  Side=Right
  b : PMIOPort  Port=5  Side=Right
  c : PMIOPort  Port=6  Side=Right
  tag scope: Iabc_2=global, Vabc_2=global
  wires:
  Model/2 -> Kv/1
  Model/1 -> Kv1/1
  Kv/1 -> Mode I/1
  Kv1/1 -> Mode V/1
  Mode I/1 -> [Iabc_2]
  Mode V/1 -> [Vabc_2]
  connections:
  Model/RConn3 -- c/RConn1
  Model/RConn1 -- a/RConn1
  Model/RConn2 -- b/RConn1
  Model/LConn3 -- C/RConn1
  Model/LConn1 -- A/RConn1
  Model/LConn2 -- B/RConn1

== system IEEE_9bus_4/SM_System/Bus_3 13.8 KV ==
  Kv : Gain  Gain=Ki  SaturateOnIntegerOverflow=on  OutDataTypeStr=Inherit: Same as input  ParamDataTypeStr=Inherit: Same as input
  Kv1 : Gain  Gain=Kv  SaturateOnIntegerOverflow=on  OutDataTypeStr=Inherit: Same as input  ParamDataTypeStr=Inherit: Same as input
  Mode I : spsVIMeasurementModel/Complex
  Mode V : spsVIMeasurementModel/Complex
  Model : spsVIMeasurementModel/VI_phase  SystemSampleTime=-1
  A : PMIOPort  Port=1  Side=Left
  B : PMIOPort  Port=2  Side=Left
  C : PMIOPort  Port=3  Side=Left
  a : PMIOPort  Port=4  Side=Right
  b : PMIOPort  Port=5  Side=Right
  c : PMIOPort  Port=6  Side=Right
  tag scope: Iabc_3=global, Vabc_3=global
  wires:
  Model/2 -> Kv/1
  Model/1 -> Kv1/1
  Kv/1 -> Mode I/1
  Kv1/1 -> Mode V/1
  Mode I/1 -> [Iabc_3]
  Mode V/1 -> [Vabc_3]
  connections:
  Model/RConn3 -- c/RConn1
  Model/RConn1 -- a/RConn1
  Model/RConn2 -- b/RConn1
  Model/LConn3 -- C/RConn1
  Model/LConn1 -- A/RConn1
  Model/LConn2 -- B/RConn1
